simulink model "rotationCount"  (R2022b)
settings: Solver=ode45  StartTime=0.0  StopTime=10.0  RelTol=1e-3  EnableMultiTasking=on
PreLoadFcn:
  | % Input data
  | load crankSpeedData
settings Model: Creator=jrivitus  LastModifiedBy=bensweet
settings SolverCC: AlgebraicLoopSolver=TrustRegion
settings DataIOCC: ExternalInput=[t,crank_speed]  LimitDataPoints=on  LoadExternalInput=on  SaveFormat=Array  ReturnWorkspaceOutputs=off
settings OptimizationCC: ExpressionDepthLimit=2147483647  LifeSpan=inf
settings DebuggingCC: UnconnectedInputMsg=warning  UnconnectedOutputMsg=warning  UnconnectedLineMsg=warning  PregeneratedLibrarySubsystemCodeDiagnostic=none  SFMachineParentedDataDiag=warning
settings HardwareCC: ProdBitPerPointer=32  ProdBitPerSizeT=32  ProdBitPerPtrDiffT=32  ProdLargestAtomicFloat=None  ProdIntDivRoundTo=Undefined  ProdEndianess=Unspecified  ProdWordSize=32  ProdHWDeviceType=32-bit Generic
settings ModelReferenceCC: EnableRefExpFcnMdlSchedulingChecks=on  PropagateSignalLabelsOutOfModel=off
settings SFSimCC: SimUseLocalCustomCode=off
settings RTWCC: RTWUseLocalCustomCode=off  DLArmComputeVersion=19.05
settings CodeAppCC: StateflowObjectComments=on
settings GRTTargetCC: TargetLangStandard=C89/C90 (ANSI)  CombineOutputUpdateFcns=off  GRTInterface=on
settings ConfigComp: CovMetricSettings=dw  CovSaveCumulativeToWorkspaceVar=on  CovSaveSingleToWorkspaceVar=on  CovExternalEMLEnable=off  CovSFcnEnable=off

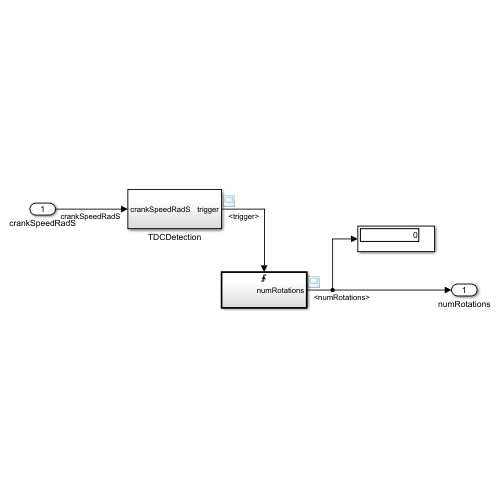
[thumbnail: Simulink's stored preview of the top-level diagram]
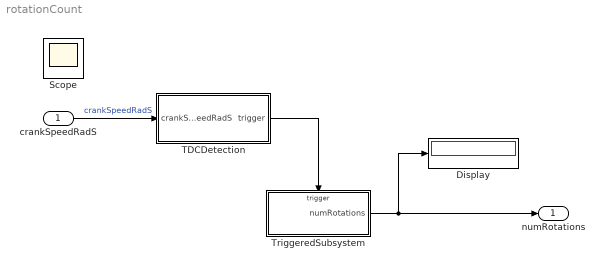
== system rotationCount ==
  crankSpeedRadS : Inport
  Display : Display
  TDCDetection : Subsystem
  TriggeredSubsystem : Subsystem  TreatAsAtomicUnit=on
  numRotations : Outport  VectorParamsAs1DForOutWhenUnconnected=off
  Scope : Scope
  wires:
  TDCDetection/1(trigger) -> TriggeredSubsystem/Trigger
  TriggeredSubsystem/1(numRotations) -> numRotations/1, Display/1
  crankSpeedRadS/1 -> TDCDetection/1(crankSpeedRadS)  "crankSpeedRadS"

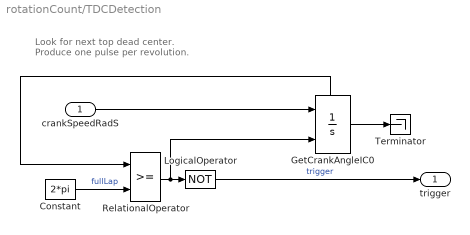
== system rotationCount/TDCDetection ==
  note: Look for next top dead center.
      | Produce one pulse per revolution.
  crankSpeedRadS : Inport
  Constant : Constant  Value=2*pi
  GetCrankAngleIC0 : Integrator  ExternalReset=rising  ShowStatePort=on
  LogicalOperator : Logic  Operator=NOT  AllPortsSameDT=off  OutDataTypeStr=boolean
  RelationalOperator : RelationalOperator
  Terminator : Terminator
  trigger : Outport  InitialOutput=0  VectorParamsAs1DForOutWhenUnconnected=off
  wires:
  crankSpeedRadS/1 -> GetCrankAngleIC0/1
  RelationalOperator/1 -> LogicalOperator/1, GetCrankAngleIC0/2
  Constant/1 -> RelationalOperator/2  "fullLap"
  GetCrankAngleIC0/State -> RelationalOperator/1
  GetCrankAngleIC0/1 -> Terminator/1
  LogicalOperator/1 -> trigger/1  "trigger"

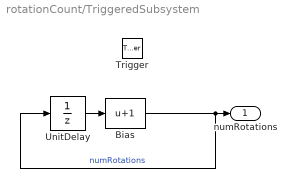
== system rotationCount/TriggeredSubsystem ==
  Trigger : TriggerPort  VariantControl=Variant  PortDimensions=1
  Bias : Bias  Bias=1  SaturateOnIntegerOverflow=off
  UnitDelay : UnitDelay  SampleTime=-1  HasFrameUpgradeWarning=on
  numRotations : Outport  VectorParamsAs1DForOutWhenUnconnected=off
  wires:
  UnitDelay/1 -> Bias/1
  Bias/1 -> numRotations/1, UnitDelay/1  "numRotations"
